simulink model "servomotor_model"  (R2014a)
settings: Solver=ode23tb  StartTime=0.0  StopTime=10  FixedStep=0.001
PreLoadFcn:
  | load spe_servomotor.mat
values from neighbouring files (symbols this model uses):
  J = 3.2284e-6    (= 3.2284e-06)    [servo.m]
undefined symbols (not defined in the file or in its folder): Jd, Km, La, Ra, sigbuilder_block, x0
libraries: powerlib x11, driveline x8, simulink x2
settings Model: Creator=The MathWorks Inc.  LastModifiedBy=JinilGondalia
settings SolverCC: SolverResetMethod=Robust
settings DataIOCC: LimitDataPoints=off  SignalLoggingSaveFormat=ModelDataLogs  SaveOutput=off  SignalLogging=off  SaveTime=off
settings OptimizationCC: ExpressionDepthLimit=2147483647  InitFltsAndDblsToZero=on  OptimizeModelRefInitCode=on  LifeSpan=1
settings DebuggingCC: AlgebraicLoopMsg=none  ArtificialAlgebraicLoopMsg=none  SaveWithParameterizedLinksMsg=none  UnderspecifiedInitializationDetection=Classic  SignalResolutionControl=TryResolveAllWithWarning  SolverPrmCheckMsg=none  MultiTaskDSMMsg=warning  MultiTaskCondExecSysMsg=none  FcnCallInpInsideContextMsg=UseLocalSettings  StateNameClashWarn=warning
settings SFSimCC: SimParseCustomCode=off
settings RTWCC: SystemTargetFile=ert.tlc  GenCodeOnly=on  TemplateMakefile=ert_default_tmf  Description=RTW Embedded Coder (no auto configuration)  ProcessScript=ert_make_rtw_hook  IncludeERTFirstTime=on
settings CodeAppCC: IgnoreCustomStorageClasses=off  CustomSymbolStrType=$N$R$M  InternalIdentifier=Classic
settings ERTTargetCC: TargetFcnLib=ansi_tfl_tmw.mat  ParMdlRefBuildCompliant=on  CompOptLevelCompliant=on  ConcurrentExecutionCompliant=on  ERTFirstTimeCompliant=on  SupportContinuousTime=on  SupportNonInlinedSFcns=on  ModelStepFunctionPrototypeControlCompliant=on  CPPClassGenCompliant=on  InlinedParameterPlacement=Hierarchical  ERTCustomFileTemplate=example_file_process.tlc

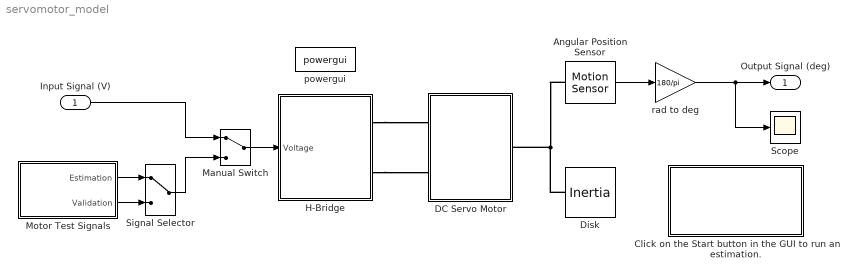
== system servomotor_model ==
  Input Signal (V) : Inport
  Angular Position Sensor : driveline/Sensors & Actuators/Motion Sensor  Angle=on  x0=x0*pi/180  Velocity=off  Acceleration=off
  Click on the Start button in the GUI to run an estimation. : Subsystem
      settings: OpenFcn=speload('spe_servomotor_project', 'Project - DCServoMotor', 'DC Motor Estimation');
      mask Display: disp('Parameter Estimation\nGUI with preloaded data')
  DC Servo Motor : Subsystem
      mask Display: image('spe_servomotor_motor.jpg')
  Disk : driveline/Solver & Inertias/Inertia  PortType=*  BlockClass=Inertia  PhysicalDomain=driveline_domain  I=Jd  Ip=[]  Iv=[]  ShowLeft=off  ShowRight=on
  H-Bridge : Subsystem
      mask Display: image('spe_servomotor_hbridge.jpg')
  Manual Switch : ManualSwitch
  Motor Test Signals : Subsystem  Tag=STV Subsys  LoadFcn=sigbuilder_block('load');  StartFcn=sigbuilder_block('start');  StopFcn=sigbuilder_block('stop');  ClipboardFcn=sigbuilder_block('clipboard');  mask(Sigbuilder block){}
      mask help: Sigbuilder GUI
      mask init:
      | if ~strcmp(get_param(bdroot(gcbh),'SimulationStatus'),'stopped') tuvar = sigbuilder_block('maskInit'); end
      settings: CopyFcn=sigbuilder_block('copy');  DeleteFcn=sigbuilder_block('delete');  ModelCloseFcn=sigbuilder_block('modelClose');  PreSaveFcn=sigbuilder_block('preSave');  PauseFcn=sigbuilder_block('pause')  ContinueFcn=sigbuilder_block('continue')  NameChangeFcn=sigbuilder_block('namechange');  OpenFcn=sigbuilder_block('open',[435.657 122.903 520.59 399.685 ]);  CloseFcn=sigbuilder_block('close');
      mask Display: plot(0,0,100,100,[10,10,40,40,10],[80,20,20,80,80],[40,10],[50,50], [40,27,10],[65,72,56],[40,25,25,10],[28,28,43,43]);
  Scope : Scope
      settings: TimeRange=10  YMin=-40  YMax=40
  Signal Selector : ManualSwitch
  powergui : powerlib/powergui  SimulationMode=Continuous  SolverType=Tustin  SampleTime=50e-6  frequency=60  SPID=off  DisableSnubberDevices=off  DisableRonSwitches=off  DisableVfSwitches=off  SwTol=0  Interpol=off  DisplayEquations=off  Ts=0  methode=off  frequencyindice=0  Pbase=100e6  ErrMax=1e-4  Iterations=50  UnitsV=kV  UnitsW=MW  FunctionMessages=off  echomessages=off  HookPort=off  EnableUseOfTLC=off  x0status=blocks  RestoreLinks=warning  ResistiveCurrentMeasurement=off  Frange=[0:2:500]  Ylog=off  Xlog=on  ShowGrid=off  save=off  variable=ZData  structure=0  ZoomFFT=on  StartTime=0.0  cycles=1  DisplayStyle=1  fundamental=60  FreqAxis=off  MaxFrequency=1000  frequencyindicesteady=1  RmsSteady=1  display=off
  rad to deg : Gain  Gain=180/pi
  Output Signal (deg) : Outport
  wires:
  Input Signal (V)/1 -> Manual Switch/1
  Manual Switch/1 -> H-Bridge/1(Voltage)
  rad to deg/1 -> Output Signal (deg)/1, Scope/1
  Angular Position Sensor/1 -> rad to deg/1
  Motor Test Signals/1(Estimation) -> Signal Selector/1
  Motor Test Signals/2(Validation) -> Signal Selector/2
  Signal Selector/1 -> Manual Switch/2
  connections:
  H-Bridge/RConn1 -- DC Servo Motor/LConn1
  H-Bridge/RConn2 -- DC Servo Motor/LConn2
  Angular Position Sensor/LConn1 -- Disk/RConn1 -- DC Servo Motor/RConn1

== system servomotor_model/Click on the Start button in the GUI to run an estimation. ==

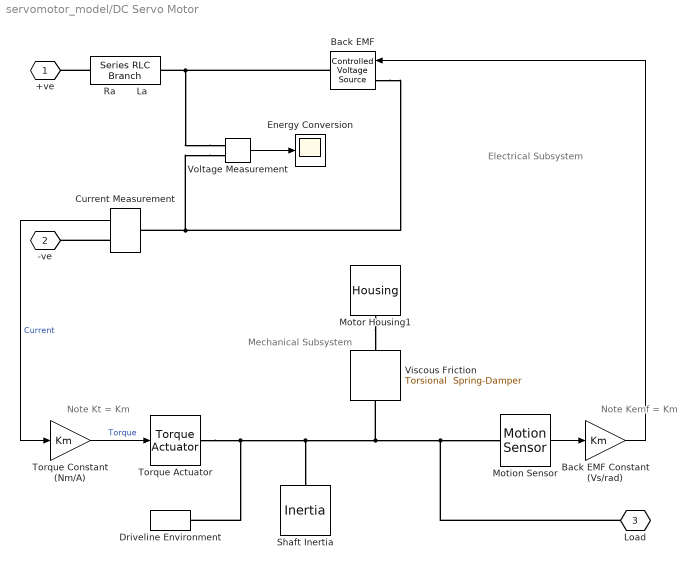
== system servomotor_model/DC Servo Motor ==
  note: Electrical
      | Subsystem
  note: Mechanical
      | Subsystem
  note: Note
      | Kt = Km
  note: Note
      | Kemf = Km
  Back EMF : powerlib/Electrical Sources/Controlled Voltage Source  Initialize=off  Source_Type=AC  Amplitude=0  Phase=0  Frequency=0  Measurements=None
  Back EMF Constant (Vs/rad) : Gain  Gain=Km
  Current Measurement : powerlib/Measurements/Current Measurement  PhasorSimulation=off  OutputType=Complex  PSBequivalent=0
  Driveline Environment : driveline/Solver & Inertias/Driveline Environment  PortType=p1  BlockClass=Solver  PhysicalDomain=driveline_domain  SimulationMode=Dynamics  ModeIteration=off  DefaultClutchVelocityTolerance=1e-3  DefaultUseAutoClutchVelocityTolerance=on
  Energy Conversion : Scope
      settings: TimeRange=10  YMin=-0.04  YMax=0.06  SaveName=ScopeData11
  Motion Sensor : driveline/Sensors & Actuators/Motion Sensor  Angle=off  x0=0  Velocity=on  Acceleration=off
  Motor Housing1 : driveline/Solver & Inertias/Housing
  Ra       La : powerlib/Elements/Series RLC Branch  LConnTagsString=__new0  RConnTagsString=__new0  BranchType=RL  Resistance=Ra  Inductance=La  SetiL0=off  InitialCurrent=0  Capacitance=1.0  Setx0=off  InitialVoltage=0  Measurements=None
  Shaft Inertia : driveline/Solver & Inertias/Inertia  PortType=p1  BlockClass=Inertia  PhysicalDomain=driveline_domain  I=J  Ip=[]  Iv=[]  ShowLeft=off  ShowRight=on
  Torque Actuator : driveline/Sensors & Actuators/Torque Actuator
  Torque Constant (Nm/A) : Gain  Gain=Km
  Viscous Friction : driveline/Dynamic Elements/Torsional  Spring-Damper  k=0  c=B  x0=0  Backlash=0
  Voltage Measurement : powerlib/Measurements/Voltage Measurement  PhasorSimulation=off  OutputType=Complex  PSBequivalent=0
  +ve : PMIOPort  Tag=PMCPort  Port=1  Side=Left
  -ve : PMIOPort  Tag=PMCPort  Port=2  Side=Left
  Load : PMIOPort  Port=3  Side=Right
  wires:
  Torque Constant (Nm/A)/1 -> Torque Actuator/1  "Torque"
  Current Measurement/1 -> Torque Constant (Nm/A)/1  "Current"
  Back EMF Constant (Vs/rad)/1 -> Back EMF/1
  Voltage Measurement/1 -> Energy Conversion/1
  Motion Sensor/1 -> Back EMF Constant (Vs/rad)/1
  connections:
  Ra       La/LConn1 -- +ve/RConn1
  Viscous Friction/LConn1 -- Driveline Environment/LConn1 -- Torque Actuator/RConn1 -- Shaft Inertia/RConn1 -- Motion Sensor/LConn1 -- Load/RConn1
  Current Measurement/RConn1 -- -ve/RConn1
  Voltage Measurement/LConn1 -- Ra       La/RConn1 -- Back EMF/RConn1
  Voltage Measurement/LConn2 -- Current Measurement/LConn1 -- Back EMF/LConn1
  Motor Housing1/RConn1 -- Viscous Friction/RConn1

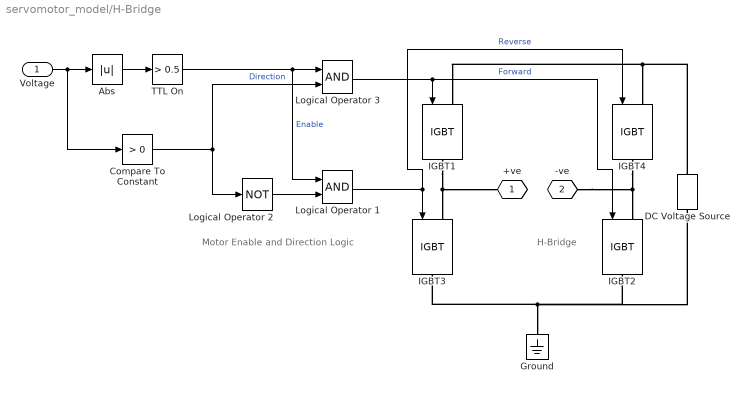
== system servomotor_model/H-Bridge ==
  note: Motor Enable and Direction Logic
  note: H-Bridge
  Voltage : Inport
  Abs : Abs
  Compare To Constant : simulink/Logic and Bit Operations/Compare To Constant  relop=>  const=0  OutDataTypeStr=boolean  ZeroCross=off
  DC Voltage Source : powerlib/Electrical Sources/DC Voltage Source  Amplitude=6.2  Measurements=None
  Ground : powerlib/Elements/Ground  LConnTagsString=a
  IGBT{1..4} (4 alike) : powerlib/Power Electronics/IGBT  Ron=0.001  Lon=1e-6  Vf=1  Tf=1e-6  Tt=2e-6  IC=0  Rs=1e5  Cs=inf  Measurements=off
  Logical Operator 1 : Logic  AllPortsSameDT=off  OutDataTypeStr=boolean
  Logical Operator 2 : Logic  Operator=NOT  AllPortsSameDT=off  OutDataTypeStr=boolean
  Logical Operator 3 : Logic  AllPortsSameDT=off  OutDataTypeStr=boolean
  TTL On : simulink/Logic and Bit Operations/Compare To Constant  relop=>  const=0.5  OutDataTypeStr=boolean  ZeroCross=off
  +ve : PMIOPort  Tag=PMCPort  Port=1  Side=Right
  -ve : PMIOPort  Tag=PMCPort  Port=2  Side=Right
  wires:
  TTL On/1 -> Logical Operator 3/1, Logical Operator 1/1  "Enable"
  Logical Operator 1/1 -> IGBT3/1, IGBT4/1  "Reverse"
  Logical Operator 3/1 -> IGBT2/1, IGBT1/1  "Forward"
  Compare To Constant/1 -> Logical Operator 3/2, Logical Operator 2/1  "Direction"
  Logical Operator 2/1 -> Logical Operator 1/2
  Voltage/1 -> Abs/1, Compare To Constant/1
  Abs/1 -> TTL On/1
  connections:
  IGBT2/RConn1 -- DC Voltage Source/LConn1 -- IGBT3/RConn1 -- Ground/LConn1
  DC Voltage Source/RConn1 -- IGBT1/LConn1 -- IGBT4/LConn1
  IGBT1/RConn1 -- +ve/RConn1 -- IGBT3/LConn1
  IGBT4/RConn1 -- IGBT2/LConn1 -- -ve/RConn1

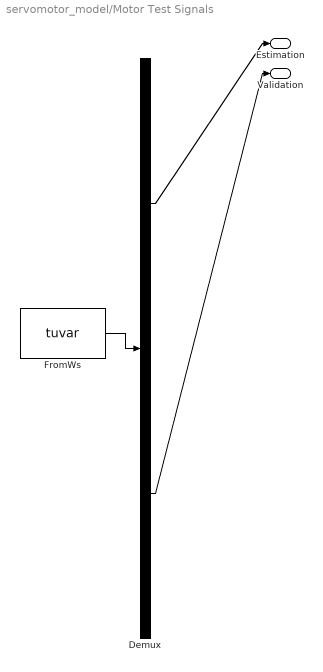
== system servomotor_model/Motor Test Signals ==
  Demux : Demux  Tag=STV Demux  Outputs=2
  FromWs : FromWorkspace  Tag=STV FromWs  VariableName=tuvar  SampleTime=0
      SigBuilderData=|
      | dataSet.timeRange = [0 5]
      | dataSet.name = 'Test Signals'
      | sbobj.Groups.Name = 'Test Signals'
      | sbobj.Groups.Signals(1).Name = 'Estimation'
      | sbobj.Groups.Signals(1).XData = [0 0.25 0.25 0.5 0.5 0.75 0.75 1 1 1.25 1.25 1.5 1.5 1.75 1.75 2 2 2.25 2.25 2.5 2.5 2.75 2.75 3 3 3.25 3.25 3.5 3.5 3.75 3.75 4 4 4.25 4.25 4.5 4.5 4.75 4.75 5]
      | sbobj.Groups.Signals(1).YData = [1 1 -1 -1 1 1 -1 -1 1 1 -1 -1 1 1 -1 -1 1 1 -1 -1 1 1 -1 -1 1 1 -1 -1 1 1 -1 -1 1 1 -1 -1 1 1 -1 -1]
      | sbobj.Groups.Signals(2).Name = 'Validation'
      | sbobj.Groups.Signals(2).XData = [0 0.75 0.75 1 1 1.5 1.5 1.75 1.75 5]
      | sbobj.Groups.Signals(2).YData = [0 0 1 1 -1 -1 1 1 0 0]
      | sbobj.Groups.TimeRange = [0 5]
  Estimation : Outport  Tag=STV Outport
  Validation : Outport  Tag=STV Outport  Port=2
  wires:
  Demux/1 -> Estimation/1
  FromWs/1 -> Demux/1
  Demux/2 -> Validation/1
